simulink model "model_2heaters_reg"  (R2023b)
settings: Solver=FixedStepAuto  StartTime=0.0  StopTime=2500  FixedStep=0.5  RelTol=1e-3
values from neighbouring files (symbols this model uses):
  C2K = 273.15    [dual_heater1.m]    (also in dual_heater_linear.m; one_heater1.m; variables.m)
  K1 = (U*A)/(m*cp)    (= 0.0035)    [dual_heater1.m]    (also in dual_heater_linear.m; one_heater1.m = 0.006)
  K2 = (eps*sig*A)/(m*cp)    (= 9.9225e-12)    [dual_heater1.m]    (also in dual_heater_linear.m; one_heater1.m = 1.701e-11)
  K3 = (U*As)/(m*cp)    (= 0.0025)    [dual_heater1.m]    (also in dual_heater_linear.m)
  K4 = (eps*sig*As)/(m*cp)    (= 7.0875e-12)    [dual_heater1.m]    (also in dual_heater_linear.m)
  Ku1 = alfa/(m*cp)    (= 0.005)    [dual_heater1.m]    (also in dual_heater_linear.m; one_heater1.m)
  Ku2 = alfa2/(m*cp)    (= 0.00375)    [dual_heater1.m]    (also in dual_heater_linear.m)
  T0 = T0 + C2K    (= 296.15)    [dual_heater1.m]    (also in dual_heater_linear.m; one_heater1.m)
  T_inf = T_inf + C2K    (= 296.15)    [dual_heater1.m]    (also in dual_heater_linear.m; one_heater1.m; variables.m)
libraries: simulink x1, slpidlib x1
settings Model: Creator=Ondra  LastModifiedBy=Ondra

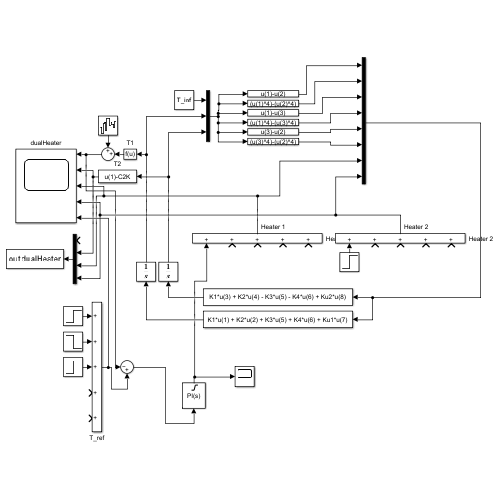
[thumbnail: Simulink's stored preview of the top-level diagram]
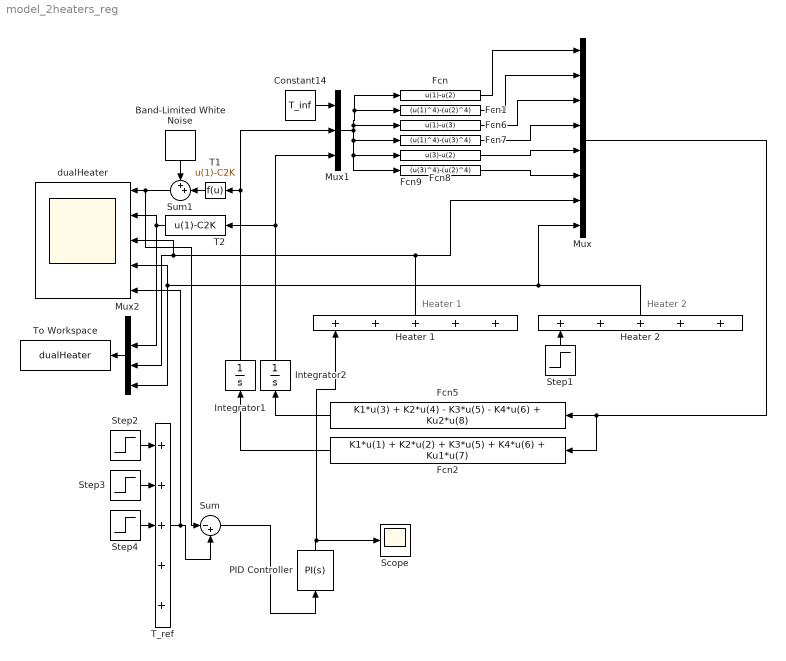
== system model_2heaters_reg ==
  note: Heater 1
  note: Heater 2
  Band-Limited White Noise : simulink/Sources/Band-Limited White Noise  Cov=1  Ts=0.5  seed=[23341]
  Constant14 : Constant  Value=T_inf
  Fcn : Fcn  Expr=u(1)-u(2)
  Fcn1 : Fcn  Expr=(u(1)^4)-(u(2)^4)
  Fcn2 : Fcn  Expr=K1*u(1) + K2*u(2) + K3*u(5) + K4*u(6) + Ku1*u(7)
  Fcn5 : Fcn  Expr=K1*u(3) + K2*u(4) - K3*u(5) - K4*u(6) + Ku2*u(8)
  Fcn6 : Fcn  Expr=u(1)-u(3)
  Fcn7 : Fcn  Expr=(u(1)^4)-(u(3)^4)
  Fcn8 : Fcn  Expr=u(3)-u(2)
  Fcn9 : Fcn  Expr=(u(3)^4)-(u(2)^4)
  Heater 1 : Sum  Inputs=+++++
  Heater 2 : Sum  Inputs=+++++
  Integrator1 : Integrator  InitialCondition=T0
  Integrator2 : Integrator  InitialCondition=T0
  Mux : Mux  Inputs=8
  Mux1 : Mux  Inputs=3
  Mux2 : Mux
  PID Controller : slpidlib/PID Controller  Controller=PI  Form=Parallel  TimeDomain=Continuous-time  UseExternalTs=off  SampleTime=-1  IntegratorMethod=Forward Euler  FilterMethod=Forward Euler  ControllerParametersSource=internal  P=0.8  I=0.02  UseKiTs=off  D=0  N=100  UseFilter=on  TunerSelectOption=Transfer Function Based (PID Tuner App)  InitialConditionSource=internal  InitialConditionForIntegrator=0  InitialConditionForFilter=0  DifferentiatorICPrevScaledInput=0  ExternalReset=none  TrackingMode=off  Kt=1  LimitOutput=on  SatLimitsSource=internal  UpperSaturationLimit=100  LowerSaturationLimit=0  LinearizeAsGain=on  AntiWindupMode=none  Kb=1  LimitIntegrator=off  UpperIntegratorSaturationLimit=inf  LowerIntegratorSaturationLimit=-inf  POutMin=[]  POutMax=[]  IOutMin=[]  IOutMax=[]  DOutMin=[]  DOutMax=[]  NOutMin=[]  NOutMax=[]  SumOutMin=[]  SumOutMax=[]  SaturationOutMin=[]  SaturationOutMax=[]  PParamMin=[]  PParamMax=[]  IParamMin=[]  IParamMax=[]  DParamMin=[]  DParamMax=[]  NParamMin=[]  NParamMax=[]  KbParamMin=[]  KbParamMax=[]  KtParamMin=[]  KtParamMax=[]  KbOutMin=[]  KbOutMax=[]  KtOutMin=[]  KtOutMax=[]  IntegratorOutMin=[]  IntegratorOutMax=[]  FilterOutMin=[]  FilterOutMax=[]  SumI1OutMin=[]  SumI1OutMax=[]  SumI2OutMin=[]  SumI2OutMax=[]  SumI3OutMin=[]  SumI3OutMax=[]  SumI4OutMin=[]  SumI4OutMax=[]  SumDOutMin=[]  SumDOutMax=[]  DifferentiatorOutMin=[]  DifferentiatorOutMax=[]  FilterDiffOutCoefMin=[]  FilterDiffOutCoefMax=[]  ReciprocalOutMin=[]  ReciprocalOutMax=[]  SumDenOutMin=[]  SumDenOutMax=[]  SumNumOutMin=[]  SumNumOutMax=[]  DivideOutMin=[]  DivideOutMax=[]  UdiffTsProdOutMin=[]  UdiffTsProdOutMax=[]  NTsProdOutMin=[]  NTsProdOutMax=[]  UintegralTsProdOutMin=[]  UintegralTsProdOutMax=[]  UngainTsProdOutMin=[]  UngainTsProdOutMax=[]  ClampingZeroOutDataTypeStr=Inherit: Inherit via back propagation  ClampingZeroOutMin=[]  ClampingZeroOutMax=[]  FilterDenConstantOutDataTypeStr=Inherit: Inherit via back propagation  FilterDenConstantOutMin=[]  FilterDenConstantOutMax=[]  PCopyOutDataTypeStr=Inherit: Inherit via back propagation  PCopyOutMin=[]  PCopyOutMax=[]  NCopyOutDataTypeStr=Inherit: Inherit via back propagation  NCopyOutMin=[]  NCopyOutMax=[]  IntegratorContinuousStateAttributes=''  IntegratorStateMustResolveToSignalObject=off  IntegratorRTWStateStorageClass=Auto  FilterContinuousStateAttributes=''  FilterStateMustResolveToSignalObject=off  FilterRTWStateStorageClass=Auto  ParallelPVariant=InternalParameters  IdealPVariant=Disabled  IVariant=InternalParameters  DVariant=Disabled  IntegratorVariant=Continuous  SatVariant=Enabled  AWVariant=Passthrough  PCopyVariant=Disabled  TRVariant=Disabled  FdbkBlocksVariant=Forward  IdealPFdbkVariant=Disabled  SatFdbkVariant=Disabled  DerivativeFilterVariant=Disabled  NVariant=Disabled  NCopyVariant=Disabled_SignalSpec  FilterICVariant=Disabled  IntegratorICVariant=InternalICs  ExternalResetVariant=Disabled  TRSumVariant=Passthrough  SumFdbkVariant=Disabled  SumVariant=Sum_PI  TsampFilterVariant=InternalTs  TsampNgainVariant=Passthrough  TsampIntegralVariant=Disabled_SignalSpec  ExternalSaturationOutDataTypeStr=Inherit: Same as second input
  Scope : Scope
  Step1 : Step  Time=0  After=40  SampleTime=0
  Step2 : Step  Time=0  After=70  SampleTime=0
  Step3 : Step  Time=1000  After=-10  SampleTime=0
  Step4 : Step  Time=2000  After=20  SampleTime=0
  Sum : Sum  Inputs=|-+
  Sum1 : Sum  Inputs=++|
  T1 : Fcn  Expr=u(1)-C2K
  T2 : Fcn  Expr=u(1)-C2K
  T_ref : Sum  Inputs=+++++
  To Workspace : ToWorkspace  VariableName=dualHeater  SaveFormat=Timeseries  SampleTime=-1
  dualHeater : Scope  NumInputPorts=5
  wires:
  Heater 1/1 -> Mux/7, Mux2/3, dualHeater/3
  Integrator1/1 -> Mux1/2, T1/1
  Mux1/1 -> Fcn/1, Fcn1/1, Fcn6/1, Fcn9/1, Fcn8/1, Fcn7/1
  Fcn2/1 -> Integrator1/1
  Fcn/1 -> Mux/1
  T1/1 -> Sum1/2
  Fcn1/1 -> Mux/2
  Constant14/1 -> Mux1/1
  PID Controller/1 -> Heater 1/1, Scope/1
  Integrator2/1 -> Mux1/3, T2/1
  Heater 2/1 -> Mux/8, dualHeater/4, Mux2/4
  Step1/1 -> Heater 2/1
  T2/1 -> Mux2/2, dualHeater/2
  Fcn6/1 -> Mux/3
  Fcn7/1 -> Mux/4
  Fcn8/1 -> Mux/5
  Fcn9/1 -> Mux/6
  Mux/1 -> Fcn2/1, Fcn5/1
  Fcn5/1 -> Integrator2/1
  Mux2/1 -> To Workspace/1
  T_ref/1 -> dualHeater/5, Sum/2
  Sum/1 -> PID Controller/1
  Step2/1 -> T_ref/1
  Step3/1 -> T_ref/2
  Step4/1 -> T_ref/3
  Band-Limited White Noise/1 -> Sum1/1
  Sum1/1 -> Sum/1, dualHeater/1
